simulink model "Particle_Formation"  (R2024b)
settings: Solver=ode4  StartTime=0.0  StopTime=200  FixedStep=0.001  RelTol=1e-3
settings Model: Creator=Omar  LastModifiedBy=Omar
settings SolverCC: ZeroCrossAlgorithm=Adaptive
settings DebuggingCC: IgnoredZcDiagnostic=none

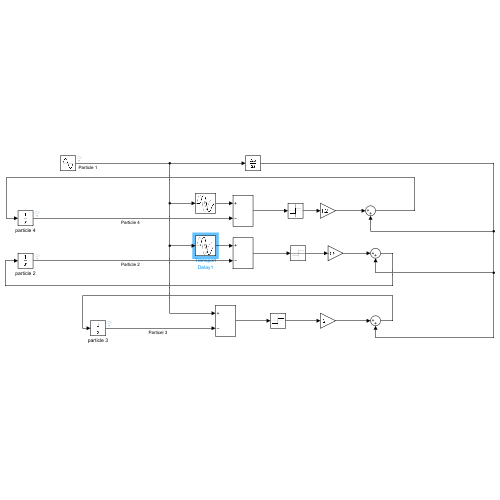
[thumbnail: Simulink's stored preview of the top-level diagram]
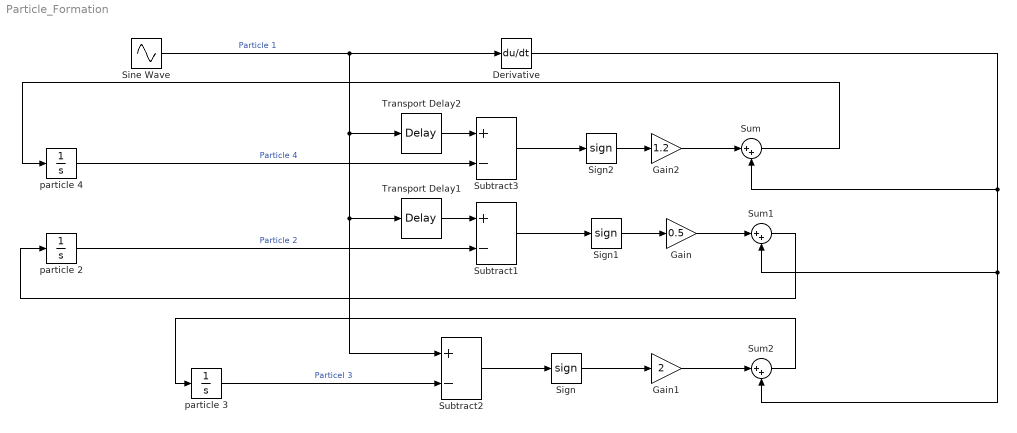
== system Particle_Formation ==
  Derivative : Derivative
  Gain : Gain  Gain=0.5
  Gain1 : Gain  Gain=2
  Gain2 : Gain  Gain=1.2
  Sign : Signum
  Sign1 : Signum
  Sign2 : Signum
  Sine Wave : Sin  SampleTime=0
  Subtract1 : Sum  Inputs=+-
  Subtract2 : Sum  Inputs=+-
  Subtract3 : Sum  Inputs=+-
  Sum : Sum  Inputs=|++
  Sum1 : Sum  Inputs=|++
  Sum2 : Sum  Inputs=|++
  Transport Delay1 : TransportDelay  DelayTime=0.2
  Transport Delay2 : TransportDelay
  particle 2 : Integrator  InitialCondition=1
  particle 3 : Integrator  InitialCondition=50
  particle 4 : Integrator  InitialCondition=1
  wires:
  particle 2/1 -> Subtract1/2  "Particle 2"
  particle 3/1 -> Subtract2/2  "Particel 3"
  Subtract2/1 -> Sign/1
  Subtract1/1 -> Sign1/1
  Sign1/1 -> Gain/1
  Sign/1 -> Gain1/1
  particle 4/1 -> Subtract3/2  "Particle 4"
  Sine Wave/1 -> Derivative/1, Transport Delay2/1, Transport Delay1/1, Subtract2/1  "Particle 1"
  Gain2/1 -> Sum/1
  Derivative/1 -> Sum/2, Sum2/2, Sum1/2
  Sum/1 -> particle 4/1
  Sign2/1 -> Gain2/1
  Subtract3/1 -> Sign2/1
  Transport Delay1/1 -> Subtract1/1
  Transport Delay2/1 -> Subtract3/1
  Gain/1 -> Sum1/1
  Sum1/1 -> particle 2/1
  Gain1/1 -> Sum2/1
  Sum2/1 -> particle 3/1
